simulink model "SkywalkerX8_Control"  (R2018a)
settings: Solver=FixedStepAuto  StartTime=0.0  StopTime=120  FixedStep=0.01  RelTol=1e-3
undefined symbols (not defined in the file): sigbuilder_block, SkywalkerX8
libraries: simulink x5, simulink_extras x3
(part 2 of 2)

== system SkywalkerX8_Control/Autopilot/Gain Scheduled Controller Phi/PDF Controller Phi 2DOF ==
  u : Inport
  P : Inport  Port=2
  D : Inport  Port=3
  N : Inport  Port=4
  Integrator : Integrator
  POut : Product
  Product : Product
  Product1 : Product
  Sum : Sum  Inputs=|+-
  Sum2 : Sum
  y : Outport  InitialOutput=0
  wires:
  Sum2/1 -> y/1
  N/1 -> Product1/1
  Product1/1 -> Sum2/2, Integrator/1
  Sum/1 -> Product1/2
  POut/1 -> Sum2/1
  D/1 -> Product/2
  u/1 -> Product/1, POut/2  "u"
  Integrator/1 -> Sum/2
  Product/1 -> Sum/1
  P/1 -> POut/1

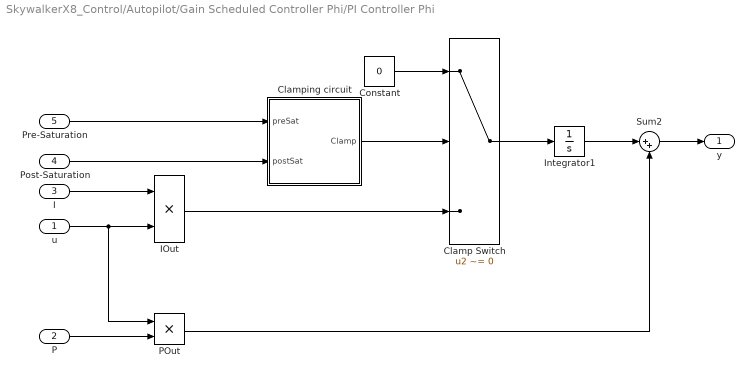
== system SkywalkerX8_Control/Autopilot/Gain Scheduled Controller Phi/PI Controller Phi ==
  u : Inport
  P : Inport  Port=2
  I : Inport  Port=3
  Post-Saturation : Inport  Port=4
  Pre-Saturation : Inport  Port=5
  Clamp Switch : Switch  Criteria=u2 ~= 0
  Clamping circuit : Subsystem
  Constant : Constant  Value=0
  IOut : Product  DisableCoverage=on
  Integrator1 : Integrator  InitialCondition=SkywalkerX8.InitialConditions.da  IgnoreLimit=on
  POut : Product
  Sum2 : Sum  Inputs=|++
  y : Outport  InitialOutput=0
  wires:
  IOut/1 -> Clamp Switch/3
  Clamp Switch/1 -> Integrator1/1
  Sum2/1 -> y/1
  Pre-Saturation/1 -> Clamping circuit/1(preSat)
  Post-Saturation/1 -> Clamping circuit/2(postSat)
  Clamping circuit/1(Clamp) -> Clamp Switch/2
  Constant/1 -> Clamp Switch/1
  Integrator1/1 -> Sum2/1
  POut/1 -> Sum2/2
  P/1 -> POut/2
  u/1 -> POut/1, IOut/2
  I/1 -> IOut/1

== system SkywalkerX8_Control/Autopilot/Gain Scheduled Controller Theta/DF Controller Theta ==
  N : Inport
  D : Inport  Port=2
  du/dt : Inport  Port=3
  Integrator : Integrator
  Product : Product
  Product1 : Product
  Sum : Sum  Inputs=|+-
  de* : Outport
  wires:
  Integrator/1 -> de*/1, Sum/2  "de*"
  Product1/1 -> Integrator/1  "Nde*_e"
  du/dt/1 -> Product/2
  D/1 -> Product/1
  Sum/1 -> Product1/2  "de*_e"
  N/1 -> Product1/1
  Product/1 -> Sum/1

== system SkywalkerX8_Control/Autopilot/Gain Scheduled Controller Theta/PDF Controller Theta 2DOF ==
  u : Inport
  P : Inport  Port=2
  D : Inport  Port=3
  N : Inport  Port=4
  Integrator : Integrator  InitialCondition=SkywalkerX8.InitialConditions.ThetaController.RefController.Derivative
  POut : Product
  Product : Product
  Product1 : Product
  Sum : Sum  Inputs=|+-
  Sum2 : Sum
  y : Outport  InitialOutput=0
  wires:
  Sum2/1 -> y/1
  N/1 -> Product1/1
  Product1/1 -> Sum2/2, Integrator/1
  Sum/1 -> Product1/2
  POut/1 -> Sum2/1
  D/1 -> Product/2
  u/1 -> Product/1, POut/2  "u"
  Integrator/1 -> Sum/2
  Product/1 -> Sum/1
  P/1 -> POut/1

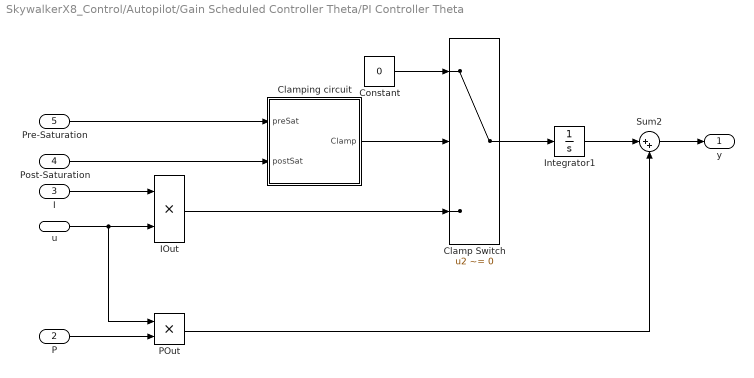
== system SkywalkerX8_Control/Autopilot/Gain Scheduled Controller Theta/PI Controller Theta ==
  u : Inport
  P : Inport  Port=2
  I : Inport  Port=3
  Post-Saturation : Inport  Port=4
  Pre-Saturation : Inport  Port=5
  Clamp Switch : Switch  Criteria=u2 ~= 0
  Clamping circuit : Subsystem
  Constant : Constant  Value=0
  IOut : Product  DisableCoverage=on
  Integrator1 : Integrator  InitialCondition=SkywalkerX8.InitialConditions.ThetaController.Integrator  IgnoreLimit=on
  POut : Product
  Sum2 : Sum  Inputs=|++
  y : Outport  InitialOutput=0
  wires:
  IOut/1 -> Clamp Switch/3
  Clamp Switch/1 -> Integrator1/1
  Sum2/1 -> y/1
  Pre-Saturation/1 -> Clamping circuit/1(preSat)
  Post-Saturation/1 -> Clamping circuit/2(postSat)
  Clamping circuit/1(Clamp) -> Clamp Switch/2
  Constant/1 -> Clamp Switch/1
  Integrator1/1 -> Sum2/1
  POut/1 -> Sum2/2
  P/1 -> POut/2
  u/1 -> POut/1, IOut/2
  I/1 -> IOut/1

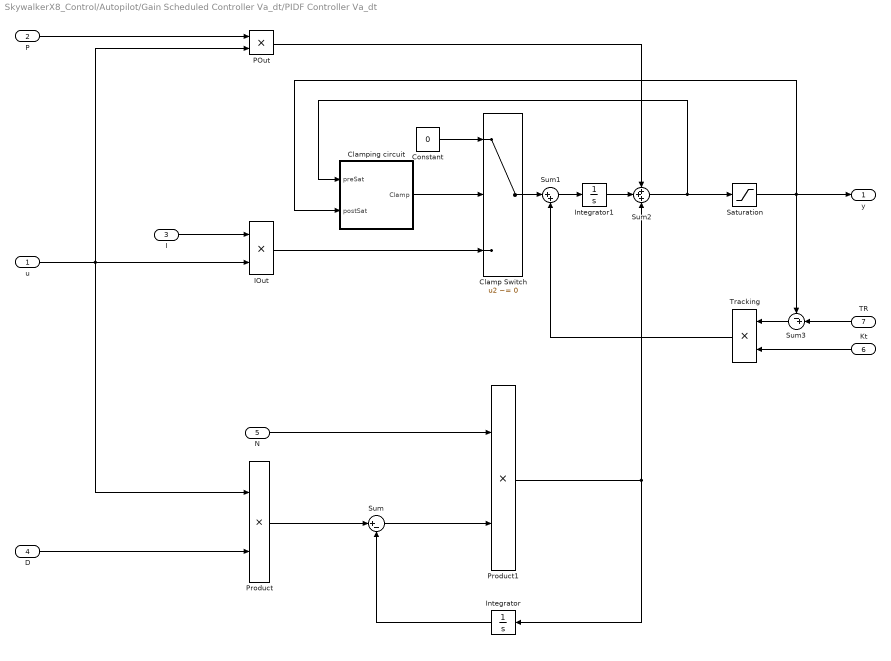
== system SkywalkerX8_Control/Autopilot/Gain Scheduled Controller Va_dt/PIDF Controller Va_dt ==
  u : Inport
  P : Inport  Port=2
  I : Inport  Port=3
  D : Inport  Port=4
  N : Inport  Port=5
  Kt : Inport  Port=6
  TR : Inport  Port=7
  Clamp Switch : Switch  Criteria=u2 ~= 0
  Clamping circuit : Subsystem
  Constant : Constant  Value=0
  IOut : Product  DisableCoverage=on
  Integrator : Integrator
  Integrator1 : Integrator  InitialCondition=SkywalkerX8.InitialConditions.VaDtController.Integrator  IgnoreLimit=on
  POut : Product
  Product : Product
  Product1 : Product
  Saturation : Saturate  UpperLimit=SkywalkerX8.Control.Longitudinal.VaDtController.upperSaturationDt  LowerLimit=SkywalkerX8.Control.Longitudinal.VaDtController.lowerSaturationDt
  Sum : Sum  Inputs=|+-
  Sum1 : Sum  Inputs=|++
  Sum2 : Sum  Inputs=+++
  Sum3 : Sum  Inputs=-+|
  Tracking : Product  DisableCoverage=on
  y : Outport  InitialOutput=0
  wires:
  Saturation/1 -> Clamping circuit/2(postSat), y/1, Sum3/1
  N/1 -> Product1/1
  Product1/1 -> Sum2/3, Integrator/1
  Sum2/1 -> Saturation/1, Clamping circuit/1(preSat)
  Sum/1 -> Product1/2
  POut/1 -> Sum2/1
  D/1 -> Product/2
  u/1 -> Product/1, POut/2, IOut/2
  Integrator/1 -> Sum/2
  Clamp Switch/1 -> Sum1/1
  Product/1 -> Sum/1
  Integrator1/1 -> Sum2/2
  Constant/1 -> Clamp Switch/1
  I/1 -> IOut/1
  IOut/1 -> Clamp Switch/3
  Clamping circuit/1(Clamp) -> Clamp Switch/2
  P/1 -> POut/1
  TR/1 -> Sum3/2
  Sum3/1 -> Tracking/1
  Kt/1 -> Tracking/2
  Tracking/1 -> Sum1/2
  Sum1/1 -> Integrator1/1

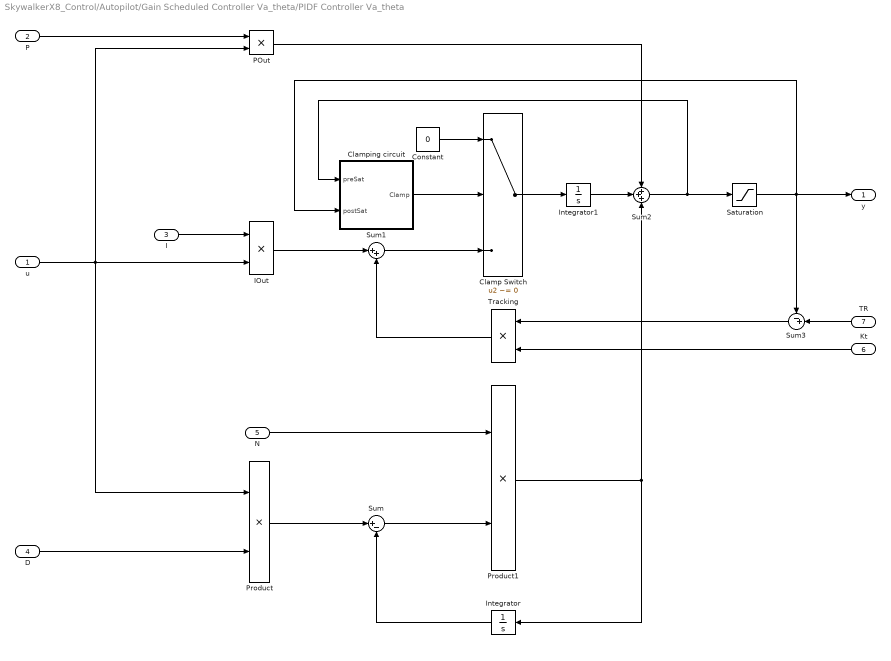
== system SkywalkerX8_Control/Autopilot/Gain Scheduled Controller Va_theta/PIDF Controller Va_theta ==
  u : Inport
  P : Inport  Port=2
  I : Inport  Port=3
  D : Inport  Port=4
  N : Inport  Port=5
  Kt : Inport  Port=6
  TR : Inport  Port=7
  Clamp Switch : Switch  Criteria=u2 ~= 0
  Clamping circuit : Subsystem
  Constant : Constant  Value=0
  IOut : Product  DisableCoverage=on
  Integrator : Integrator
  Integrator1 : Integrator  InitialCondition=-SkywalkerX8.InitialConditions.PhiThetaPsi(2)  IgnoreLimit=on
  POut : Product
  Product : Product
  Product1 : Product
  Saturation : Saturate  UpperLimit=SkywalkerX8.Control.Longitudinal.VaThetaController.upperSaturationThetaC  LowerLimit=SkywalkerX8.Control.Longitudinal.VaThetaController.lowerSaturationThetaC
  Sum : Sum  Inputs=|+-
  Sum1 : Sum  Inputs=|++
  Sum2 : Sum  Inputs=+++
  Sum3 : Sum  Inputs=-+|
  Tracking : Product  DisableCoverage=on
  y : Outport  InitialOutput=0
  wires:
  Saturation/1 -> Clamping circuit/2(postSat), y/1, Sum3/1
  N/1 -> Product1/1
  Product1/1 -> Sum2/3, Integrator/1
  Sum2/1 -> Saturation/1, Clamping circuit/1(preSat)
  Sum/1 -> Product1/2
  POut/1 -> Sum2/1
  D/1 -> Product/2
  u/1 -> Product/1, POut/2, IOut/2
  Integrator/1 -> Sum/2
  Clamp Switch/1 -> Integrator1/1
  Product/1 -> Sum/1
  Integrator1/1 -> Sum2/2
  Constant/1 -> Clamp Switch/1
  I/1 -> IOut/1
  Sum1/1 -> Clamp Switch/3
  Clamping circuit/1(Clamp) -> Clamp Switch/2
  P/1 -> POut/1
  IOut/1 -> Sum1/1
  TR/1 -> Sum3/2
  Sum3/1 -> Tracking/1
  Kt/1 -> Tracking/2
  Tracking/1 -> Sum1/2

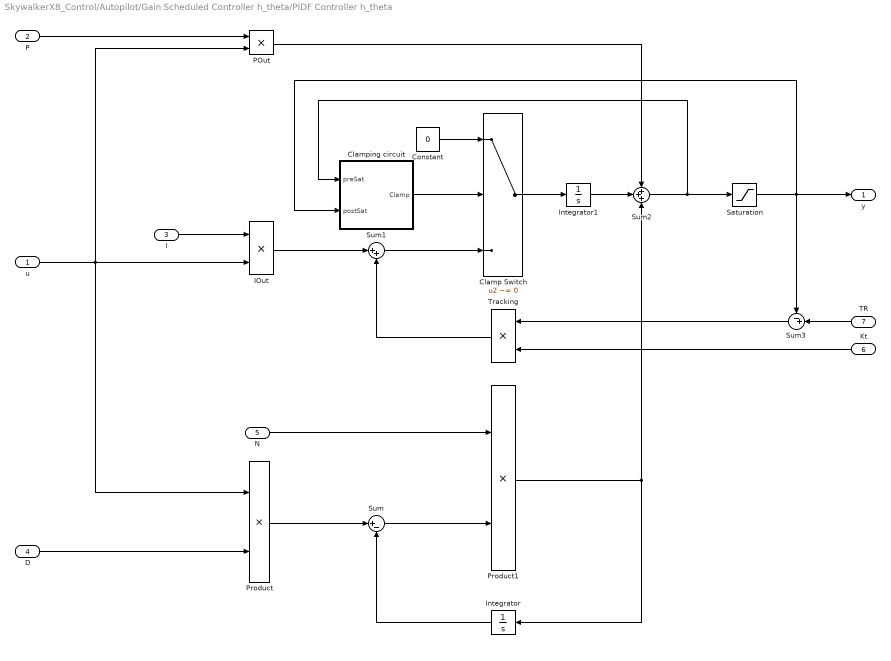
== system SkywalkerX8_Control/Autopilot/Gain Scheduled Controller h_theta/PIDF Controller h_theta ==
  u : Inport
  P : Inport  Port=2
  I : Inport  Port=3
  D : Inport  Port=4
  N : Inport  Port=5
  Kt : Inport  Port=6
  TR : Inport  Port=7
  Clamp Switch : Switch  Criteria=u2 ~= 0
  Clamping circuit : Subsystem
  Constant : Constant  Value=0
  IOut : Product  DisableCoverage=on
  Integrator : Integrator
  Integrator1 : Integrator  InitialCondition=SkywalkerX8.InitialConditions.altController.Integrator  IgnoreLimit=on
  POut : Product
  Product : Product
  Product1 : Product
  Saturation : Saturate  UpperLimit=SkywalkerX8.Control.Longitudinal.altController.upperSaturationThetaC  LowerLimit=SkywalkerX8.Control.Longitudinal.altController.lowerSaturationThetaC
  Sum : Sum  Inputs=|+-
  Sum1 : Sum  Inputs=|++
  Sum2 : Sum  Inputs=+++
  Sum3 : Sum  Inputs=-+|
  Tracking : Product  DisableCoverage=on
  y : Outport  InitialOutput=0
  wires:
  Saturation/1 -> Clamping circuit/2(postSat), y/1, Sum3/1
  N/1 -> Product1/1
  Product1/1 -> Sum2/3, Integrator/1
  Sum2/1 -> Saturation/1, Clamping circuit/1(preSat)
  Sum/1 -> Product1/2
  POut/1 -> Sum2/1
  D/1 -> Product/2
  u/1 -> Product/1, POut/2, IOut/2
  Integrator/1 -> Sum/2
  Clamp Switch/1 -> Integrator1/1
  Product/1 -> Sum/1
  Integrator1/1 -> Sum2/2
  Constant/1 -> Clamp Switch/1
  I/1 -> IOut/1
  Sum1/1 -> Clamp Switch/3
  Clamping circuit/1(Clamp) -> Clamp Switch/2
  P/1 -> POut/1
  IOut/1 -> Sum1/1
  TR/1 -> Sum3/2
  Sum3/1 -> Tracking/1
  Kt/1 -> Tracking/2
  Tracking/1 -> Sum1/2

== system SkywalkerX8_Control/Autopilot/Gain Scheduled Controller Chi/PIDF Controller Va_theta/Clamping circuit ==
  preSat : Inport  DisableCoverage=on
  postSat : Inport  DisableCoverage=on  Port=2
  Memory : Memory  DisableCoverage=on
  NotEqual : RelationalOperator  DisableCoverage=on  Operator=~=  RndMeth=Nearest  InputSameDT=on
  Clamp : Outport  DisableCoverage=on
  wires:
  postSat/1 -> NotEqual/2
  preSat/1 -> NotEqual/1
  NotEqual/1 -> Memory/1
  Memory/1 -> Clamp/1

== system SkywalkerX8_Control/Autopilot/Gain Scheduled Controller Phi/PI Controller Phi/Clamping circuit ==
  preSat : Inport  DisableCoverage=on
  postSat : Inport  DisableCoverage=on  Port=2
  Memory : Memory  DisableCoverage=on
  NotEqual : RelationalOperator  DisableCoverage=on  Operator=~=  RndMeth=Nearest  InputSameDT=on
  Clamp : Outport  DisableCoverage=on
  wires:
  postSat/1 -> NotEqual/2
  preSat/1 -> NotEqual/1
  NotEqual/1 -> Memory/1
  Memory/1 -> Clamp/1

== system SkywalkerX8_Control/Autopilot/Gain Scheduled Controller Theta/PI Controller Theta/Clamping circuit ==
  preSat : Inport  DisableCoverage=on
  postSat : Inport  DisableCoverage=on  Port=2
  Memory : Memory  DisableCoverage=on
  NotEqual : RelationalOperator  DisableCoverage=on  Operator=~=  RndMeth=Nearest  InputSameDT=on
  Clamp : Outport  DisableCoverage=on
  wires:
  postSat/1 -> NotEqual/2
  preSat/1 -> NotEqual/1
  NotEqual/1 -> Memory/1
  Memory/1 -> Clamp/1

== system SkywalkerX8_Control/Autopilot/Gain Scheduled Controller Va_dt/PIDF Controller Va_dt/Clamping circuit ==
  preSat : Inport  DisableCoverage=on
  postSat : Inport  DisableCoverage=on  Port=2
  Memory : Memory  DisableCoverage=on
  NotEqual : RelationalOperator  DisableCoverage=on  Operator=~=  RndMeth=Nearest  InputSameDT=on
  Clamp : Outport  DisableCoverage=on
  wires:
  postSat/1 -> NotEqual/2
  preSat/1 -> NotEqual/1
  NotEqual/1 -> Memory/1
  Memory/1 -> Clamp/1

== system SkywalkerX8_Control/Autopilot/Gain Scheduled Controller Va_theta/PIDF Controller Va_theta/Clamping circuit ==
  preSat : Inport  DisableCoverage=on
  postSat : Inport  DisableCoverage=on  Port=2
  Memory : Memory  DisableCoverage=on
  NotEqual : RelationalOperator  DisableCoverage=on  Operator=~=  RndMeth=Nearest  InputSameDT=on
  Clamp : Outport  DisableCoverage=on
  wires:
  postSat/1 -> NotEqual/2
  preSat/1 -> NotEqual/1
  NotEqual/1 -> Memory/1
  Memory/1 -> Clamp/1

== system SkywalkerX8_Control/Autopilot/Gain Scheduled Controller h_theta/PIDF Controller h_theta/Clamping circuit ==
  preSat : Inport  DisableCoverage=on
  postSat : Inport  DisableCoverage=on  Port=2
  Memory : Memory  DisableCoverage=on
  NotEqual : RelationalOperator  DisableCoverage=on  Operator=~=  RndMeth=Nearest  InputSameDT=on
  Clamp : Outport  DisableCoverage=on
  wires:
  postSat/1 -> NotEqual/2
  preSat/1 -> NotEqual/1
  NotEqual/1 -> Memory/1
  Memory/1 -> Clamp/1

== stateflow chart SkywalkerX8_Control/Autopilot/Altitude Control State Machine ==
  settings: executeAtInitialization=1
  state Descend_Zone
    during: dt = 0
    during: theta_c = theta_c_Va
  state Altitude_Hold_Zone
    during: dt = dt_Va
    during: theta_c = theta_c_h
  state Landing_Mode
    during: dt = 0
    during: theta_c = theta_c_h
  state Climb_Zone
    during: dt = 1.0
    during: theta_c = theta_c_Va
  state Take_Off_Zone
    during: dt = 1.0
    during: theta_c = theta_c_takeoff
  state Pre_Flight
    during: dt = dt_Va
    during: theta_c = theta_c_h
  Descend_Zone -> Landing_Mode [order 2] : [ h_c == 0 ]
  Altitude_Hold_Zone -> Descend_Zone [order 2] : [h >= (h_c + h_hold*(1+hyst_frac))]
  Descend_Zone -> Altitude_Hold_Zone [order 1] : [h < (h_c + h_hold*(1-hyst_frac))]
  Altitude_Hold_Zone -> Landing_Mode [order 3] : [ h_c == 0 ]
  Pre_Flight -> Altitude_Hold_Zone [order 1] : [PreFlightBypass]
  Climb_Zone -> Altitude_Hold_Zone [order 2] : [h >= (h_c - h_hold*(1+hyst_frac))]
  Altitude_Hold_Zone -> Climb_Zone [order 1] : [h < (h_c - h_hold*(1-hyst_frac))]
  Climb_Zone -> Landing_Mode [order 3] : [ h_c == 0 ]
  Landing_Mode -> Pre_Flight : [ h == 0 ]
  Take_Off_Zone -> Landing_Mode [order 2] : [ h_c == 0 ]
  Take_Off_Zone -> Climb_Zone [order 1] : [h >= h_takeoff*(1+hyst_frac)]
  Climb_Zone -> Take_Off_Zone [order 1] : [h < h_takeoff*(1-hyst_frac)]
  Pre_Flight -> Take_Off_Zone [order 2] : [ h_c > 0 ]
  (default) -> Pre_Flight
  data: dt_Va input; theta_c_Va input; theta_c_h input; h input; h_c input; dt output; theta_c output; h_hold parameter double; theta_c_takeoff parameter double; h_takeoff parameter double; hyst_frac parameter double; PreFlightBypass parameter
